simulink model "towTest_dualWinch"  (R2020a)
settings: Solver=FixedStepAuto  StartTime=0.0  StopTime=inf  FixedStep=Ts  RelTol=1e-3  EnableMultiTasking=on
undefined symbols (not defined in the file): encAng_trig, IO397, standard
libraries: xpcutilitieslib x52, hdlsllib x29, simulink x11, slrtlib x9, dspsigops x5, xpcseriallib x2, speedgoatlib_fpga_quadrature x2, powerlib_meascontrol x2, xpcrtudplib x2, speedgoatlib_fpga_dio x1, speedgoatlib_fpga_analog_io x1, speedgoatlib_IO581 x1
(part 1 of 2)
settings Model: Creator=MAE-VermillionLab  LastModifiedBy=MAE-VermillionLab
settings SolverCC: ConcurrentTasks=on  AutoInsertRateTranBlk=on
settings DataIOCC: SaveFormat=StructureWithTime
settings OptimizationCC: BlockReduction=off  OptimizeBlockIOStorage=off
settings HardwareCC: ProdBitPerPointer=32  ProdBitPerSizeT=32  ProdBitPerPtrDiffT=32  ProdLargestAtomicFloat=None  ProdWordSize=32  ProdLongLongMode=on  ProdHWDeviceType=Generic->32-bit x86 compatible
settings RTWCC: Description=Simulink Real-Time  SystemTargetFile=slrt.tlc  TLCOptions=-axPCMaxOverloads=30 -axPCOverLoadLen=2 -axPCStartupFlag=5  TemplateMakefile=slrt_default_tmf  CodeExecutionProfiling=on  RTWCompilerOptimization=on
settings SimulinkRealTimeCC: SupportVariableSizeSignals=on  RL32LogBufSizeModifier=1e8  xPCConcurrentTasks=on

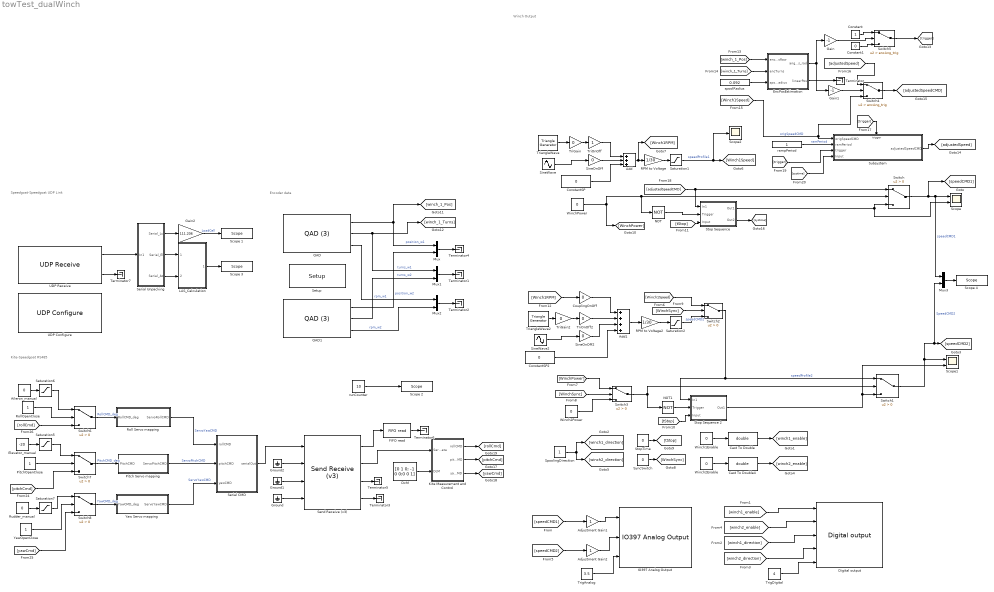
== system towTest_dualWinch ==
  note: Kite-Speedgoat RS485
  note: Speedgoat-Speedgoat UDP Link
  note: Winch Output
  note: Encoder data
  Add : Sum  Inputs=+++
  Add1 : Sum  Inputs=++++
  Adjustment Gain1 : Gain
  Adjustment Gain2 : Gain
  Aileron_manual : Constant  Value=0  OutDataTypeStr=int8
  Cast To Double : DataTypeConversion  OutDataTypeStr=double
  Cast To Double4 : DataTypeConversion  OutDataTypeStr=double
  Constant : Constant
  Constant1 : Constant  Value=0
  ConstantSP : Constant  Value=0
  ConstantSP2 : Constant  Value=0
  CouplingOnOff : Gain  Gain=0
  DcM : Constant  Value=[0 1 0; -1 0 0;0 0 1]
  Digital output : speedgoatlib_fpga_dio/Digital output  id=1  chan=[1:5]  init=[0]  reset=[0]  vectorizeInput=off  ts=Ts  pciSlot=-1  board=IO397-50k
      settings: SourceProductName=Simulink Real-Time: Speedgoat I/O Driver Library
  Elevator_manual : Constant  Value=-20  OutDataTypeStr=int8
  "EncPosEstimation " : Subsystem
  "FIFO read " : xpcseriallib/FIFO read   maxsize=1024  minsize=1  usedelimiter=off  delimiter=13  outputtype=8 bit uint null terminated  enable=off  enableout=off  sampletime=0.01
      settings: SourceProductBaseCode=XP
  Gain : Gain  Gain=-1
  Gain1 : Gain  Gain=-1
  Gain2 : Gain  Gain=111.206
  Ground : Ground
  Ground1 : Ground
  Ground2 : Ground
  IO397 Analog Output : speedgoatlib_fpga_analog_io/IO397 Analog Output  id=1  chan=[1:3]  initVal=0  resetVal=0  ts=Ts  pciSlot=-1  board=IO397-50k  span=+5 V
      settings: SourceProductName=Simulink Real-Time: Speedgoat I/O Driver Library
  "Kite Measurement and Control " : Subsystem
  LAS_Calculation : Subsystem
  Mux{,1..3} (4 alike) : Mux  Inputs=2
  NOT : Logic  Operator=NOT  IconShape=distinctive  AllPortsSameDT=off  OutDataTypeStr=boolean
  NOT1 : Logic  Operator=NOT  IconShape=distinctive  AllPortsSameDT=off  OutDataTypeStr=boolean
  "Pitch Servo mapping " : Subsystem
  PitchOpenClose : Constant
  QAD : speedgoatlib_fpga_quadrature/QAD (3)  id=1  board=IO397-50k  chan=[1]  resetOnStart=on  ts=Ts  pciSlot=-1  operatingMode=Quadrature decoder  indexControlMode=Ignore index  resolution=1x  stepsPerRevolution=[1800]  latchMode=Disabled  interpolatePosition=off  invertAB=off  showClearPositionInput=off  showClearIndexFoundInput=off  showPositionOutput=on  showTurnOutput=on  showSpeedOutput=on  showDirectionOutput=off  showIndexFoundOutput=off
      settings: SourceProductName=Simulink Real-Time: Speedgoat I/O Driver Library
  QAD1 : speedgoatlib_fpga_quadrature/QAD (3)  id=1  board=IO397-50k  chan=[2]  resetOnStart=on  ts=Ts  pciSlot=-1  operatingMode=Quadrature decoder  indexControlMode=Ignore index  resolution=1x  stepsPerRevolution=1800  latchMode=Disabled  interpolatePosition=off  invertAB=off  showClearPositionInput=off  showClearIndexFoundInput=off  showPositionOutput=on  showTurnOutput=on  showSpeedOutput=on  showDirectionOutput=off  showIndexFoundOutput=off
      settings: SourceProductName=Simulink Real-Time: Speedgoat I/O Driver Library
  RPM to Voltage : Gain  Gain=1/30
  RPM to Voltage2 : Gain  Gain=1/30
  Roll Servo mapping : Subsystem
  RollOpenClose : Constant
  Rudder_manual : Constant  Value=0  OutDataTypeStr=int8
  Saturation1 : Saturate  UpperLimit=5  LowerLimit=0
  Saturation2 : Saturate  UpperLimit=5  LowerLimit=0
  Saturation5 : Saturate  UpperLimit=30  LowerLimit=-30
  Saturation6 : Saturate  UpperLimit=30  LowerLimit=-30
  Saturation7 : Saturate  UpperLimit=30  LowerLimit=-30
  Scope : Scope  NumInputPorts=2
  Scope 1 : slrtlib/Displays and Logging/Scope   scopeno=6  scopetype=Target  autostart=on  viewmode=Numerical  formatstr='%15.6f'  grid=on  ylimits=[0,0]  nosamples=50  noprepostsamples=0  interleave=1  triggermode=FreeRun  triggersignal=1  trigsignalfromport=off  triggerlevel=0.0  triggerslope=Either  triggerscope=1  triggersample=0  filename=data.dat  mode=Lazy  writesize=512  autorestart=off  dynamicfilemode=off  maxwritefilesize=512*1024^2
  Scope 2 : slrtlib/Displays and Logging/Scope   scopeno=4  scopetype=Target  autostart=on  viewmode=Numerical  formatstr='%15.6f'  grid=on  ylimits=[0,0]  nosamples=50  noprepostsamples=0  interleave=1  triggermode=FreeRun  triggersignal=1  trigsignalfromport=off  triggerlevel=0.0  triggerslope=Either  triggerscope=1  triggersample=0  filename=data.dat  mode=Lazy  writesize=512  autorestart=off  dynamicfilemode=off  maxwritefilesize=512*1024^2
  Scope 3 : slrtlib/Displays and Logging/Scope   scopeno=5  scopetype=Target  autostart=on  viewmode=Numerical  formatstr='%15.6f'  grid=on  ylimits=[0,0]  nosamples=50  noprepostsamples=0  interleave=1  triggermode=FreeRun  triggersignal=1  trigsignalfromport=off  triggerlevel=0.0  triggerslope=Either  triggerscope=1  triggersample=0  filename=data.dat  mode=Lazy  writesize=512  autorestart=off  dynamicfilemode=off  maxwritefilesize=512*1024^2
  Scope 4 : slrtlib/Displays and Logging/Scope   scopeno=9  scopetype=Target  autostart=on  viewmode=Graphical sliding  formatstr='%15.6f'  grid=on  ylimits=[0,6]  nosamples=500  noprepostsamples=0  interleave=1  triggermode=FreeRun  triggersignal=1  trigsignalfromport=off  triggerlevel=0.0  triggerslope=Either  triggerscope=1  triggersample=0  filename=data.dat  mode=Lazy  writesize=512  autorestart=off  dynamicfilemode=off  maxwritefilesize=512*1024^2
  Scope1 : Scope  NumInputPorts=2
  Scope2 : Scope
  "Send Receive (v3) " : speedgoatlib_IO581/Send Receive (v3)   parModuleId=1  parSlot=-1  parModuleType=IO581  parTransceiver12=RS485 Half-Duplex  parTransceiver34=RS422  parTransceiver1=RS485 Half-Duplex  parAutoTurnaround1=off  parTurnaroundDelay1=0  parStandardBaud1=on  parBaudrate1=115200  parBaudDivisor1=1  parSamplingRate1=16x (standard)  parPrescale1=off  parCalcBaud1=7812500  parParity1=None  parDataBits1=8  parStopBits1=1  parTxTrigLvl1=1  parRxTrigLvl1=1  parHandshake1=none  parRtsHysteresis1=0  parXon1=17  parXoff1=19  parTxSwFifoSize1=1024  parTxSwFifoType1=8 bit uint null terminated  parRxSwFifoSize1=1024  parTransceiver2=RS485 Half-Duplex  parAutoTurnaround2=off  parTurnaroundDelay2=0  parStandardBaud2=on  parBaudrate2=115200  parBaudDivisor2=1  parSamplingRate2=16x (standard)  parPrescale2=off  parCalcBaud2=7812500  parParity2=None  parDataBits2=8  parStopBits2=1  parTxTrigLvl2=1  parRxTrigLvl2=1  parHandshake2=none  parRtsHysteresis2=0  parXon2=17  parXoff2=19  parTxSwFifoSize2=1024  parTxSwFifoType2=8 bit int null terminated  parRxSwFifoSize2=1024  parTransceiver3=RS422  parAutoTurnaround3=off  parTurnaroundDelay3=0  parStandardBaud3=on  parBaudrate3=115200  parBaudDivisor3=1  parSamplingRate3=16x (standard)  parPrescale3=off  parCalcBaud3=7812500  parParity3=None  parDataBits3=8  parStopBits3=1  parTxTrigLvl3=1  parRxTrigLvl3=8  parHandshake3=none  parRtsHysteresis3=0  parXon3=17  parXoff3=19  parTxSwFifoSize3=1024  parTxSwFifoType3=8 bit uint null terminated  parRxSwFifoSize3=1024  parTransceiver4=RS422  parAutoTurnaround4=off  parTurnaroundDelay4=0  parStandardBaud4=on  parBaudrate4=115200  parBaudDivisor4=1  parSamplingRate4=16x (standard)  parPrescale4=off  parCalcBaud4=7812500  parParity4=None  parDataBits4=8  parStopBits4=1  parTxTrigLvl4=1  parRxTrigLvl4=1  parHandshake4=none  parRtsHysteresis4=0  parXon4=17  parXoff4=19  parTxSwFifoSize4=1024  parTxSwFifoType4=8 bit uint null terminated  parRxSwFifoSize4=1024
      settings: SourceProductName=Simulink Real-Time: Speedgoat Library
  Serial CMD : Subsystem
  Serial Unpacking : Subsystem
  Setup : speedgoatlib_fpga/Setup/Setup  board=IO397-50k  id=1  device_id=1  frontIO=None  rearIO=None  bitstreamFile=init.mat  rev=1.0  timestamp_string=21/04/20 11:41:53  fpgaFreq=75 MHz  fpgaTick=13.33 ns  ProgSpiFlash=off  ProgBPIFlash=off  pciSlot=-1  PullRPort0=pull-up 3.3V  VioPort0=3.3V  PullRPort1=pull-up 3.3V  VioPort1=3.3V  PullRPort2=pull-up 3.3V  VioPort2=3.3V  PullRPort3=pull-up 3.3V  VioPort3=3.3V  PullRPort4=pull-up 3.3V  VioPort4=3.3V  PullRPort5=pull-up 3.3V  VioPort5=3.3V  PullRPort6=pull-up 3.3V  VioPort6=3.3V  PullRPort15=pull-up 3.3V  PullRPort31=pull-up 3.3V  PullRPort47=pull-up 3.3V  PullRPort63=pull-up 3.3V
      settings: SourceProductName=Simulink Real-Time: Speedgoat Library
  SineOnOff : Gain  Gain=0
  SineOnOff2 : Gain  Gain=0
  SineWave : Sin  Amplitude=0  Frequency=2*pi  SampleTime=0
  SineWave2 : Sin  Amplitude=0  Frequency=2*pi  SampleTime=0
  SpoolingDirection : Constant
  "Stop Sequence " : Subsystem
  Stop Sequence 2 : Subsystem
  StopTime : Constant  Value=0
  Subsystem : Subsystem
  Switch{,1..3,6..8} (7 alike) : Switch  Criteria=u2 > Threshold
  Switch4 : Switch  Criteria=u2 > Threshold  Threshold=encAng_trig
  Switch5 : Switch  Criteria=u2 > Threshold  Threshold=encAng_trig
  SyncSwitch : Constant  Value=0
  Terminator{,1..7} (8 alike) : Terminator
  TriGain : Gain  Gain=0
  TriGain2 : Gain  Gain=0
  TriOnOff : Gain
  TriOnOff2 : Gain  Gain=0
  TriangleWave : powerlib_meascontrol/Pulse & Signal Generators/Triangle Generator  Freq=1  Phase=90  Ts=0
  TriangleWave2 : powerlib_meascontrol/Pulse & Signal Generators/Triangle Generator  Freq=1  Phase=90  Ts=0
  TrigAnalog : Constant  Value=3.5
  TrigDigital : Constant  Value=4
  UDP Configure : xpcrtudplib/UDP Configure  Priority=-1  IpAddress=30.30.30.1  SubnetMask=255.255.255.0  Gateway=0.0.0.0  PciBus=15  PciSlot=0  PciFunction=0  ID=1  tune=0  disable=off  enableMulticast=off  MulticastIpAddress={}  MulticastMask={}
      settings: SourceProductBaseCode=XP
  UDP Receive : xpcrtudplib/UDP Receive  ipAddressVal=30.30.30.1  localPort=25001  rcvWidth=8  rcvFmAny=off  fmAddress=30.30.30.2  rcvMulticast=off  multicastAddress={}  maxUDPQueue=8  sampleTime=Ts
  Winch1Enable : Constant  Value=0
  Winch2Enable : Constant  Value=0
  Winch2Power : Constant  Value=0
  WinchPower : Constant  Value=0
  Yaw Servo mapping : Subsystem
  YawOpenClose : Constant
  rampPeriod : Constant
  runCounter : Constant  Value=10
  spoolRadius : Constant  Value=0.092
  wires:
  Switch/1 -> [speedCMD1], Mux3/1, Scope/1  "speedCMD1"
  WinchPower/1 -> NOT/1, Switch/2, [WinchPower]
  NOT/1 -> "Stop Sequence "/2(Trigger)
  Saturation1/1 -> Scope2/1, [Winch1Speed]  "speedProfile1"
  [speedCMD1] -> Adjustment Gain1/1
  Adjustment Gain1/1 -> IO397 Analog Output/1
  [winch1_enable] -> Digital output/1
  Cast To Double/1 -> [winch1_enable]
  Winch1Enable/1 -> Cast To Double/1
  ConstantSP/1 -> Add/3
  Add/1 -> [Winch1RPM], RPM to Voltage/1
  SineWave/1 -> SineOnOff/1
  [winch1_direction] -> Digital output/3
  Stop Sequence 2/1(Out1) -> Switch1/3, Scope1/2
  Switch1/1 -> Mux3/2, [speedCMD2], Scope1/1  "SpeedCMD2"
  SpoolingDirection/1 -> [winch1_direction], [winch2_direction]
  Switch3/1 -> NOT1/1, Switch1/2
  Cast To Double4/1 -> [winch2_enable]
  Winch2Enable/1 -> Cast To Double4/1
  Switch2/1 -> Stop Sequence 2/1(In1), Switch1/1  "speedProfile2"
  Adjustment Gain2/1 -> IO397 Analog Output/2
  [speedCMD2] -> Adjustment Gain2/1
  [winch2_enable] -> Digital output/2
  [winch2_direction] -> Digital output/4
  TriangleWave/1 -> TriGain/1
  TriGain/1 -> TriOnOff/1
  TriOnOff/1 -> Add/1
  SineOnOff/1 -> Add/2
  RPM to Voltage/1 -> Saturation1/1
  TriangleWave2/1 -> TriGain2/1
  RPM to Voltage2/1 -> Saturation2/1
  Add1/1 -> RPM to Voltage2/1
  SineWave2/1 -> SineOnOff2/1
  TriGain2/1 -> TriOnOff2/1
  TriOnOff2/1 -> Add1/2
  SineOnOff2/1 -> Add1/3
  Saturation2/1 -> Switch2/3  "speedCMD2"
  [Winch1Speed] -> Switch2/1
  SyncSwitch/1 -> [WinchSync]
  [WinchSync] -> Switch2/2
  "Stop Sequence "/1(Out1) -> Scope/2, Switch/3
  StopTime/1 -> [tStop]
  [tStop] -> "Stop Sequence "/3(Input)
  [tStop] -> Stop Sequence 2/3(Input)
  NOT1/1 -> Stop Sequence 2/2(Trigger)
  [WinchPower] -> Switch3/1
  Winch2Power/1 -> Switch3/3
  [WinchSync] -> Switch3/2
  [Winch1RPM] -> CouplingOnOff/1
  ConstantSP2/1 -> Add1/4
  CouplingOnOff/1 -> Add1/1
  QAD1/1 -> Mux/2  "position_w2"
  QAD/1 -> [winch_1_Pos], Mux/1  "position_w1"
  QAD/2 -> [winch_1_Turns], Mux1/1  "turns_w1"
  QAD1/2 -> Mux1/2  "turns_w2"
  QAD/3 -> Mux2/1  "rpm_w1"
  QAD1/3 -> Mux2/2  "rpm_w2"
  Mux3/1 -> Scope 4/1
  [winch_1_Pos] -> "EncPosEstimation "/1(encPosRaw)
  [winch_1_Turns] -> "EncPosEstimation "/2(encTurns)
  spoolRadius/1 -> "EncPosEstimation "/3(spoolRadius)
  "EncPosEstimation "/2(linearPos) -> Terminator/1
  "EncPosEstimation "/1(angPos_rad) -> Gain/1, Gain1/1
  [Winch1Speed] -> Switch4/3, Subsystem/1(origSpeedCMD)  "origSpeedCMD"
  Constant/1 -> Switch5/1
  Constant1/1 -> Switch5/3
  rampPeriod/1 -> Subsystem/2(ramPeriod)  "ramPeriod"
  Subsystem/1(adjustedSpeedCMD) -> [adjustedSpeed]
  [trigger] -> Subsystem/Trigger
  [adjustedSpeedCMD] -> "Stop Sequence "/1(In1), Switch/1
  Switch4/1 -> [adjustedSpeedCMD]
  Gain/1 -> Switch5/2
  Gain1/1 -> Switch4/2
  [adjustedSpeed] -> Switch4/1
  Switch5/1 -> [trigger]
  [trigger] -> Subsystem/3(trigger)
  "Stop Sequence "/2(Out2) -> [systime]
  [systime] -> Subsystem/4(Input)
  Mux1/1 -> Terminator1/1
  Mux2/1 -> Terminator2/1
  Mux/1 -> Terminator4/1
  DcM/1 -> "Kite Measurement and Control "/2(DcM)
  Serial CMD/1(serialOut) -> "Send Receive (v3) "/1
  "Kite Measurement and Control "/1(rollCMD) -> [rollCmd]
  "Send Receive (v3) "/2 -> "Kite Measurement and Control "/1(SerialData)
  "Send Receive (v3) "/1 -> "FIFO read "/1
  Ground2/1 -> "Send Receive (v3) "/2
  "Kite Measurement and Control "/3(yawCMD) -> [yawCmd]
  Ground1/1 -> "Send Receive (v3) "/3
  "FIFO read "/1 -> Terminator6/1
  "Kite Measurement and Control "/2(pitchCMD) -> [pitchCmd]
  Ground/1 -> "Send Receive (v3) "/4
  "Send Receive (v3) "/4 -> Terminator3/1
  "Send Receive (v3) "/3 -> Terminator5/1
  Serial Unpacking/2(Serial_El) -> LAS_Calculation/1(Serial_El)
  UDP Receive/2 -> Terminator7/1
  Serial Unpacking/3(Serial_Az) -> LAS_Calculation/2(Serial_Az)
  UDP Receive/1 -> Serial Unpacking/1(In1)
  Serial Unpacking/1(Serial_Lc) -> Gain2/1
  LAS_Calculation/1(Output) -> Scope 3/1
  Gain2/1 -> Scope 1/1  "LoadCell"
  "Pitch Servo mapping "/1(ServoPitchCMD) -> Serial CMD/2(pitchCMD)  "ServoPitchCMD"
  Yaw Servo mapping/1(ServoYawCMD) -> Serial CMD/3(yawCMD)  "ServoYawCMD"
  Roll Servo mapping/1(ServoRollCMD) -> Serial CMD/1("rollCMD ")  "ServoYawCMD"
  [rollCmd] -> Switch6/3
  [yawCmd] -> Switch8/3
  Aileron_manual/1 -> Saturation6/1
  [pitchCmd] -> Switch7/3
  Elevator_manual/1 -> Saturation5/1
  Saturation6/1 -> Switch6/1
  Switch8/1 -> Yaw Servo mapping/1(YawCMD_deg)  "YawCMD_deg"
  Switch6/1 -> Roll Servo mapping/1(RollCMD_deg)  "RollCMD_deg"
  RollOpenClose/1 -> Switch6/2
  Rudder_manual/1 -> Saturation7/1
  Switch7/1 -> "Pitch Servo mapping "/1(PitchCMD)  "PitchCMD_deg"
  Saturation7/1 -> Switch8/1
  PitchOpenClose/1 -> Switch7/2
  YawOpenClose/1 -> Switch8/2
  Saturation5/1 -> Switch7/1
  TrigAnalog/1 -> IO397 Analog Output/3
  TrigDigital/1 -> Digital output/5
  runCounter/1 -> Scope 2/1

== system towTest_dualWinch/EncPosEstimation  ==
  encPosRaw : Inport
  encTurns : Inport  Port=2
  spoolRadius : Inport  Port=3
  Add1 : Sum
  Cast To Double : DataTypeConversion  OutDataTypeStr=double
  Gain : Gain  Gain=(2*pi)/1800
  Gain1 : Gain  Gain=1800
  Product : Product
  angPos_rad : Outport
  linearPos : Outport  Port=2
  wires:
  Gain/1 -> angPos_rad/1, Product/1  "angPos_rad"
  Cast To Double/1 -> Add1/1
  Add1/1 -> Gain/1
  Gain1/1 -> Add1/2
  Product/1 -> linearPos/1  "linearPos"
  encTurns/1 -> Gain1/1
  spoolRadius/1 -> Product/2
  encPosRaw/1 -> Cast To Double/1

== system towTest_dualWinch/Kite Measurement and Control  ==
  SerialData : Inport
  DcM : Inport  Port=2
  Bus Selector : BusSelector  OutputSignals=rollCmd,pitchCmd,yawCmd
  Controller1 : Subsystem  mask{ctrlSurfDefMax=45, pitchKP=1, yawKP=1, rollKP=1}
      mask prompts: ctrlSurfDefMax "Max Ctrlsurf def"; pitchKP "pitch Kp"; yawKP "yaw Kp"; rollKP "roll Kp"
  "Euler setpoints " : Subsystem  mask{EulerSP=[0 0 0]}
      mask prompts: EulerSP "Euler Setpoints"
  "Kite Measurements " : Subsystem
  rollCMD : Outport
  pitchCMD : Outport  Port=2
  yawCMD : Outport  Port=3
  wires:
  "Kite Measurements "/1(kiteMeasure) -> Controller1/2(kiteMeasure)  "kiteMeasure"
  Bus Selector/3 -> yawCMD/1  "<yawCmd>"
  Controller1/1(Cmd) -> Bus Selector/1
  Bus Selector/2 -> pitchCMD/1  "<pitchCmd>"
  Bus Selector/1 -> rollCMD/1  "<rollCmd>"
  SerialData/1 -> "Kite Measurements "/1(In1)
  DcM/1 -> "Kite Measurements "/2(Input)
  "Euler setpoints "/1(setPoints) -> Controller1/1(setPoints)  "setPoints"

== system towTest_dualWinch/LAS_Calculation ==
  Serial_El : Inport
  Serial_Az : Inport  Port=2
  Add2 : Sum
  Add3 : Sum
  Az_deg_calib : Constant  Value=-343.5468
  Constant : Constant  Value=360
  Constant2 : Constant  Value=360
  El_deg_calib : Constant  Value=-243.544
  Gain : Gain  Gain=360/8192
  Gain1 : Gain  Gain=360/8192
  Gain2 : Gain  Gain=pi/180
  Gain3 : Gain  Gain=pi/180
  Gain4 : Gain  Gain=180/pi
  Gain5 : Gain  Gain=180/pi
  LAS Measurement Corrections : MATLAB Function  TreatAsAtomicUnit=on
  Mod : Math  Operator=mod  SaturateOnIntegerOverflow=on
  Mod1 : Math  Operator=mod  SaturateOnIntegerOverflow=on
  Mux : Mux
  ifOutsideBounds : MATLAB Function  TreatAsAtomicUnit=on
  ifOutsideBounds1 : MATLAB Function  TreatAsAtomicUnit=on
  Output : Outport
  wires:
  Gain/1 -> Mod/1
  Constant2/1 -> Mod1/2
  Constant/1 -> Mod/2
  Mod/1 -> Add2/1
  Serial_Az/1 -> Gain1/1
  Mod1/1 -> Add3/1
  Gain1/1 -> Mod1/1
  ifOutsideBounds/1(y) -> Mux/3, Gain2/1  "El_deg"
  Add3/1 -> ifOutsideBounds1/1(u)  "Az_deg"
  Serial_El/1 -> Gain/1  "Elevation"
  Gain2/1 -> LAS Measurement Corrections/1(elev_encoder)
  Gain3/1 -> LAS Measurement Corrections/2(azi_encoder)
  LAS Measurement Corrections/2(azi) -> Gain5/1
  LAS Measurement Corrections/1(elev) -> Gain4/1
  Gain4/1 -> Mux/1  "kite_elev"
  Gain5/1 -> Mux/2  "kite_azi"
  Mux/1 -> Output/1
  Az_deg_calib/1 -> Add3/2
  El_deg_calib/1 -> Add2/2
  Add2/1 -> ifOutsideBounds/1(u)  "El_deg"
  ifOutsideBounds1/1(y) -> Gain3/1, Mux/4  "Az_deg"

== system towTest_dualWinch/Pitch Servo mapping  ==
  note: Negative gain added due to servo orientation
  PitchCMD : Inport
  Add2 : Sum
  Add3 : Sum
  "Bias " : Constant  Value=7.2
  Constant2 : Constant  Value=-0.2065
  Display : Display
  Display1 : Display
  Gain3 : Gain  Gain=2.732
  Gain4 : Gain  Gain=-1
  ServoPitchCMD : Outport
  wires:
  Add2/1 -> Add3/1
  Constant2/1 -> Add2/2
  Gain4/1 -> Gain3/1
  "Bias "/1 -> Add3/2  "PitchServoBias"
  Add3/1 -> Display/1, ServoPitchCMD/1
  PitchCMD/1 -> Display1/1, Gain4/1
  Gain3/1 -> Add2/1

== system towTest_dualWinch/Roll Servo mapping ==
  RollCMD_deg : Inport
  Add2 : Sum
  Bias : Constant  Value=0
  ServoRollCMD : Outport
  wires:
  Bias/1 -> Add2/2  "RollServoBias"
  RollCMD_deg/1 -> Add2/1
  Add2/1 -> ServoRollCMD/1

== system towTest_dualWinch/Serial CMD ==
  note: Subsystem
  "rollCMD " : Inport
  pitchCMD : Inport  Port=2
  yawCMD : Inport  Port=3
  Constant : Constant  Value=0x11  OutDataTypeStr=uint8
  Constant1 : Constant  Value=0x01  OutDataTypeStr=uint8
  Mux : Mux  Inputs=8
  Mux1 : Mux  Inputs=3
  Mux2 : Mux  Inputs=3
  Mux3 : Mux  Inputs=3
  Scope 1 : slrtlib/Displays and Logging/Scope   scopeno=3  scopetype=Target  autostart=on  viewmode=Graphical sliding  formatstr='%15.6f'  grid=on  ylimits=[-60,60]  nosamples=500  noprepostsamples=0  interleave=1  triggermode=FreeRun  triggersignal=1  trigsignalfromport=off  triggerlevel=0.0  triggerslope=Either  triggerscope=1  triggersample=0  filename=data.dat  mode=Lazy  writesize=512  autorestart=off  dynamicfilemode=off  maxwritefilesize=512*1024^2
  Scope 2 : slrtlib/Displays and Logging/Scope   scopeno=7  scopetype=Target  autostart=on  viewmode=Numerical  formatstr='%15.6f'  grid=on  ylimits=[0,100]  nosamples=50  noprepostsamples=0  interleave=1  triggermode=FreeRun  triggersignal=1  trigsignalfromport=off  triggerlevel=0.0  triggerslope=Either  triggerscope=1  triggersample=0  filename=data.dat  mode=Lazy  writesize=512  autorestart=off  dynamicfilemode=off  maxwritefilesize=512*1024^2
  Scope 3 : slrtlib/Displays and Logging/Scope   scopeno=8  scopetype=Target  autostart=on  viewmode=Numerical  formatstr='%15.6f'  grid=on  ylimits=[0,100]  nosamples=50  noprepostsamples=0  interleave=1  triggermode=FreeRun  triggersignal=1  trigsignalfromport=off  triggerlevel=0.0  triggerslope=Either  triggerscope=1  triggersample=0  filename=data.dat  mode=Lazy  writesize=512  autorestart=off  dynamicfilemode=off  maxwritefilesize=512*1024^2
  deg-to-us : Subsystem
  deg-to-us1 : Subsystem
  deg-to-us2 : Subsystem
  to2uint1 : Subsystem
  to2uint2 : Subsystem
  to2uint8 : Subsystem
  serialOut : Outport
  wires:
  pitchCMD/1 -> deg-to-us1/1(pitchCMD), Mux2/2, Mux1/2  "pitchCMD"
  Constant/1 -> Mux/2
  to2uint8/1(Out1) -> Mux/3
  to2uint8/2(Out2) -> Mux/4
  yawCMD/1 -> Mux1/3, deg-to-us2/1(In1), Mux2/3  "yawCMD"
  Mux/1 -> serialOut/1
  Mux1/1 -> Scope 1/1
  "rollCMD "/1 -> Mux1/1, deg-to-us/1(In1), Mux2/1  "rollCMD"
  to2uint1/1(Out1) -> Mux/5
  to2uint1/2(Out2) -> Mux/6
  to2uint2/1(Out1) -> Mux/7
  to2uint2/2(Out2) -> Mux/8
  deg-to-us1/1(Out1) -> to2uint1/1(" "), Mux3/2
  deg-to-us2/1(Out1) -> to2uint2/1(" "), Mux3/3
  Mux2/1 -> Scope 2/1
  Mux3/1 -> Scope 3/1
  deg-to-us/1(Out1) -> to2uint8/1(" "), Mux3/1
  Constant1/1 -> Mux/1

== system towTest_dualWinch/Serial Unpacking ==
  In1 : Inport
  Demux : Demux  Outputs=8
  Display2 : Display
  Display7 : Display
  Display8 : Display
  Subsystem : Subsystem
  Subsystem1 : Subsystem
  binary2double5 : Subsystem
  Serial_Lc : Outport
  Serial_El : Outport  Port=2
  Serial_Az : Outport  Port=3
  wires:
  Demux/6 -> Subsystem/2(In2)
  Demux/5 -> Subsystem/1(In1)
  In1/1 -> Demux/1
  Subsystem/1(Double) -> Display7/1, Serial_El/1
  Demux/8 -> Subsystem1/2(In2)
  Demux/7 -> Subsystem1/1(In1)
  Subsystem1/1(Double) -> Display8/1, Serial_Az/1
  Demux/1 -> binary2double5/1(In1)
  Demux/2 -> binary2double5/2(In2)
  Demux/3 -> binary2double5/3(In3)
  Demux/4 -> binary2double5/4(In4)
  binary2double5/1(Double) -> Display2/1, Serial_Lc/1  "Yaw Rate"

== system towTest_dualWinch/Stop Sequence  ==
  In1 : Inport
  Trigger : Inport  Port=2
  Input : Inport  Port=3
  Add : Sum  Inputs=-+
  Add1 : Sum  Inputs=+-
  Clock : Clock
  Divide : Product  Inputs=**/
  Sample and Hold : dspsigops/Sample and Hold  trig=Rising edge  initCond=0  latchinput=off
  Sample and Hold1 : dspsigops/Sample and Hold  trig=Rising edge  initCond=0  latchinput=off
  Saturation : Saturate  UpperLimit=5  LowerLimit=0
  Out1 : Outport
  Out2 : Outport  Port=2
  wires:
  Trigger/1 -> Sample and Hold1/Trigger, Sample and Hold/Trigger
  Add/1 -> Divide/2
  In1/1 -> Sample and Hold/1
  Divide/1 -> Add1/2
  Sample and Hold/1 -> Divide/1, Add1/1
  Sample and Hold1/1 -> Add/1
  Clock/1 -> Out2/1, Add/2, Sample and Hold1/1
  Add1/1 -> Saturation/1
  Saturation/1 -> Out1/1
  Input/1 -> Divide/3

== system towTest_dualWinch/Stop Sequence 2 ==
  In1 : Inport
  Trigger : Inport  Port=2
  Input : Inport  Port=3
  Add : Sum  Inputs=-+
  Add1 : Sum  Inputs=+-
  Clock : Clock
  Divide : Product  Inputs=**/
  Sample and Hold : dspsigops/Sample and Hold  trig=Rising edge  initCond=0  latchinput=off
  Sample and Hold1 : dspsigops/Sample and Hold  trig=Rising edge  initCond=0  latchinput=off
  Saturation : Saturate  UpperLimit=5  LowerLimit=0
  Out1 : Outport
  wires:
  Input/1 -> Divide/3
  Saturation/1 -> Out1/1
  Add1/1 -> Saturation/1
  Clock/1 -> Sample and Hold1/1, Add/2
  Sample and Hold1/1 -> Add/1
  Sample and Hold/1 -> Add1/1, Divide/1
  Divide/1 -> Add1/2
  In1/1 -> Sample and Hold/1
  Add/1 -> Divide/2
  Trigger/1 -> Sample and Hold/Trigger, Sample and Hold1/Trigger

== system towTest_dualWinch/Subsystem ==
  origSpeedCMD : Inport
  ramPeriod : Inport  Port=2
  trigger : Inport  Port=3
  Input : Inport  Port=4
  Trigger : TriggerPort  VariantControl=Variant  PortDimensions=1
  Add : Sum  Inputs=+-
  Add2 : Sum
  Divide : Product  Inputs=*/
  Gain : Gain  Gain=0.08
  Gain1 : Gain  Gain=1.08
  Product : Product
  Sample and Hold : dspsigops/Sample and Hold  trig=Rising edge  initCond=0  latchinput=off
  Saturation Dynamic : simulink/Discontinuities/Saturation Dynamic  OutMin=[]  OutMax=[]  OutDataTypeStr=Inherit: Same as second input  OutDataType=fixdt(1, 16)  OutScaling=2^-10  RndMeth=Zero  DoSatur=off
  adjustedSpeedCMD : Outport
  wires:
  Saturation Dynamic/1 -> adjustedSpeedCMD/1  "adjustedSpeedCMD"
  origSpeedCMD/1 -> [Winch1Speed], Gain/1
  Gain/1 -> Divide/1
  [Winch1Speed] -> Gain1/1, Saturation Dynamic/3  "origSpeedCMD"
  [Winch1Speed] -> Add2/2  "origSpeedCMD"
  Gain1/1 -> Saturation Dynamic/1
  ramPeriod/1 -> Divide/2
  Add2/1 -> Saturation Dynamic/2
  Input/1 -> [time], Sample and Hold/1
  trigger/1 -> Sample and Hold/Trigger
  Sample and Hold/1 -> [triggerTime]
  [time] -> Add/1
  [triggerTime] -> Add/2
  Divide/1 -> Product/2
  Add/1 -> Product/1
  Product/1 -> Add2/1

== system towTest_dualWinch/Yaw Servo mapping ==
  YawCMD_deg : Inport
  Add2 : Sum
  Bias : Constant  Value=0
  ServoYawCMD : Outport
  wires:
  Bias/1 -> Add2/2  "YawServoBias"
  YawCMD_deg/1 -> Add2/1
  Add2/1 -> ServoYawCMD/1

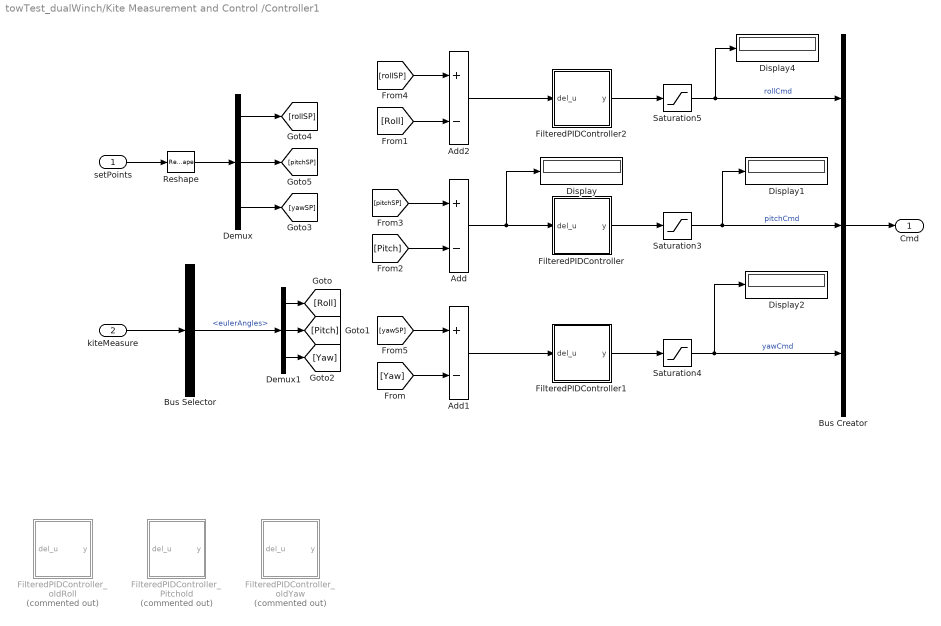
== system towTest_dualWinch/Kite Measurement and Control /Controller1 ==
  setPoints : Inport
  kiteMeasure : Inport  Port=2
  Add : Sum  Inputs=+-
  Add1 : Sum  Inputs=+-
  Add2 : Sum  Inputs=+-
  Bus Creator : BusCreator  Inputs=3
  Bus Selector : BusSelector  OutputSignals=eulerAngles
  Demux : Demux  Outputs=3
  Demux1 : Demux  Outputs=3
  Display{,1..2,4} (4 alike) : Display
  FilteredPIDController : Subsystem  mask{Kp=1, Kd=0, tau=1, Ki=0}
      mask prompts: Kp "Proportional Gain"; Kd "Derivative Gain"; tau "Time constant"; Ki "Integral Gain"
  FilteredPIDController1 : Subsystem  mask{Kp=1, Kd=0, tau=1, Ki=0}
      mask prompts: Kp "Proportional Gain"; Kd "Derivative Gain"; tau "Time constant"; Ki "Integral Gain"
  FilteredPIDController2 : Subsystem  mask{Kp=1, Kd=0, tau=1, Ki=0}
      mask prompts: Kp "Proportional Gain"; Kd "Derivative Gain"; tau "Time constant"; Ki "Integral Gain"
  FilteredPIDController_Pitchold : Subsystem  Commented=on  mask{Kp=1, Kd=0, tau=1, Ki=0}
      mask prompts: Kp "Proportional Gain"; Kd "Derivative Gain"; tau "Time constant"; Ki "Integral Gain"
  FilteredPIDController_oldRoll : Subsystem  Commented=on  mask{Kp=1, Kd=0, tau=1, Ki=0}
      mask prompts: Kp "Proportional Gain"; Kd "Derivative Gain"; tau "Time constant"; Ki "Integral Gain"
  FilteredPIDController_oldYaw : Subsystem  Commented=on  mask{Kp=1, Kd=0, tau=1, Ki=0}
      mask prompts: Kp "Proportional Gain"; Kd "Derivative Gain"; tau "Time constant"; Ki "Integral Gain"
  Reshape : Reshape  OutputDimensionality=Column vector (2-D)
  Saturation3 : Saturate  UpperLimit=30  LowerLimit=-30
  Saturation4 : Saturate  UpperLimit=30  LowerLimit=-30
  Saturation5 : Saturate  UpperLimit=30  LowerLimit=-30
  Cmd : Outport
  wires:
  [Pitch] -> Add/2
  [Yaw] -> Add1/2
  [yawSP] -> Add1/1
  Demux/3 -> [yawSP]
  [pitchSP] -> Add/1
  kiteMeasure/1 -> Bus Selector/1
  Saturation4/1 -> Display2/1, Bus Creator/3  "yawCmd"
  Saturation5/1 -> Display4/1, Bus Creator/1  "rollCmd"
  Bus Creator/1 -> Cmd/1
  Reshape/1 -> Demux/1
  setPoints/1 -> Reshape/1
  Add/1 -> FilteredPIDController/1(del_u), Display/1
  [rollSP] -> Add2/1
  [Roll] -> Add2/2
  Demux/2 -> [pitchSP]
  Demux/1 -> [rollSP]
  Bus Selector/1 -> Demux1/1  "<eulerAngles>"
  Demux1/1 -> [Roll]
  Demux1/2 -> [Pitch]
  Demux1/3 -> [Yaw]
  Saturation3/1 -> Display1/1, Bus Creator/2  "pitchCmd"
  FilteredPIDController/1(y) -> Saturation3/1
  FilteredPIDController2/1(y) -> Saturation5/1
  Add2/1 -> FilteredPIDController2/1(del_u)
  FilteredPIDController1/1(y) -> Saturation4/1
  Add1/1 -> FilteredPIDController1/1(del_u)

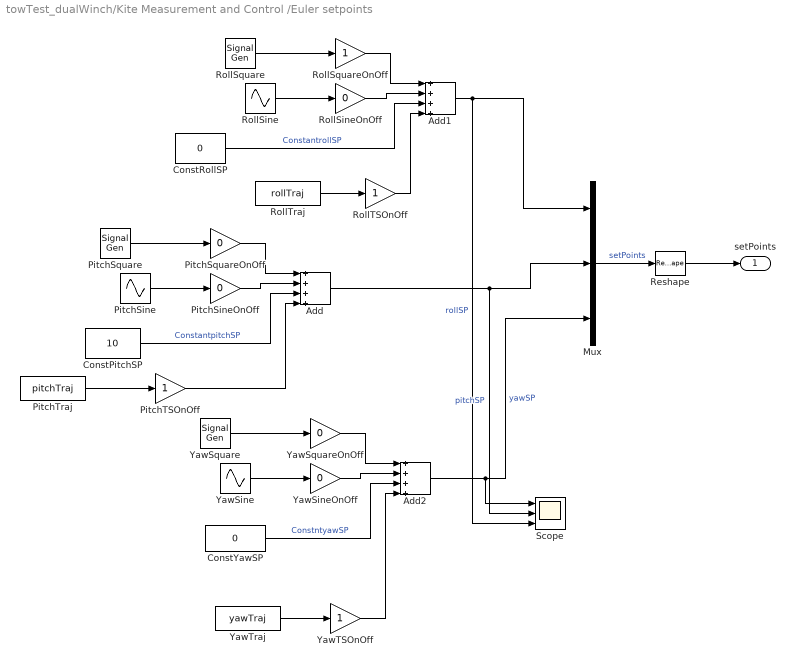
== system towTest_dualWinch/Kite Measurement and Control /Euler setpoints  ==
  Add : Sum  Inputs=++++
  Add1 : Sum  Inputs=++++
  Add2 : Sum  Inputs=++++
  ConstPitchSP : Constant  Value=10
  ConstRollSP : Constant  Value=0
  ConstYawSP : Constant  Value=0
  Mux : Mux  Inputs=3
  PitchSine : Sin  Amplitude=20  Frequency=1.5708  SampleTime=0
  PitchSineOnOff : Gain  Gain=0
  PitchSquare : SignalGenerator  WaveForm=square  Amplitude=20  Frequency=1.5708  Units=rad/sec
  PitchSquareOnOff : Gain  Gain=0
  PitchTSOnOff : Gain
  PitchTraj : FromWorkspace  VariableName=pitchTraj
  Reshape : Reshape  OutputDimensionality=Column vector (2-D)
  RollSine : Sin  Amplitude=10  Frequency=2.0944  SampleTime=0
  RollSineOnOff : Gain  Gain=0
  RollSquare : SignalGenerator  WaveForm=square  Amplitude=10  Frequency=1.0472  Units=rad/sec
  RollSquareOnOff : Gain
  RollTSOnOff : Gain
  RollTraj : FromWorkspace  VariableName=rollTraj
  Scope : Scope  NumInputPorts=3
  YawSine : Sin  Amplitude=15  Frequency=3.1416  SampleTime=0
  YawSineOnOff : Gain  Gain=0
  YawSquare : SignalGenerator  WaveForm=square  Amplitude=10  Units=rad/sec
  YawSquareOnOff : Gain  Gain=0
  YawTSOnOff : Gain
  YawTraj : FromWorkspace  VariableName=yawTraj
  setPoints : Outport
  wires:
  Mux/1 -> Reshape/1  "setPoints"
  Reshape/1 -> setPoints/1
  PitchSineOnOff/1 -> Add/2
  PitchSine/1 -> PitchSineOnOff/1
  PitchSquareOnOff/1 -> Add/1
  PitchSquare/1 -> PitchSquareOnOff/1
  ConstPitchSP/1 -> Add/3  "ConstantpitchSP"
  RollSineOnOff/1 -> Add1/2
  RollSquareOnOff/1 -> Add1/1
  RollSine/1 -> RollSineOnOff/1
  RollSquare/1 -> RollSquareOnOff/1
  ConstRollSP/1 -> Add1/3  "ConstantrollSP"
  YawSineOnOff/1 -> Add2/2
  YawSquareOnOff/1 -> Add2/1
  YawSine/1 -> YawSineOnOff/1
  YawSquare/1 -> YawSquareOnOff/1
  ConstYawSP/1 -> Add2/3  "ConstntyawSP"
  Add2/1 -> Scope/1, Mux/3  "yawSP"
  Add/1 -> Scope/2, Mux/2  "pitchSP"
  Add1/1 -> Scope/3, Mux/1  "rollSP"
  RollTSOnOff/1 -> Add1/4
  RollTraj/1 -> RollTSOnOff/1
  PitchTSOnOff/1 -> Add/4
  YawTSOnOff/1 -> Add2/4
  PitchTraj/1 -> PitchTSOnOff/1
  YawTraj/1 -> YawTSOnOff/1

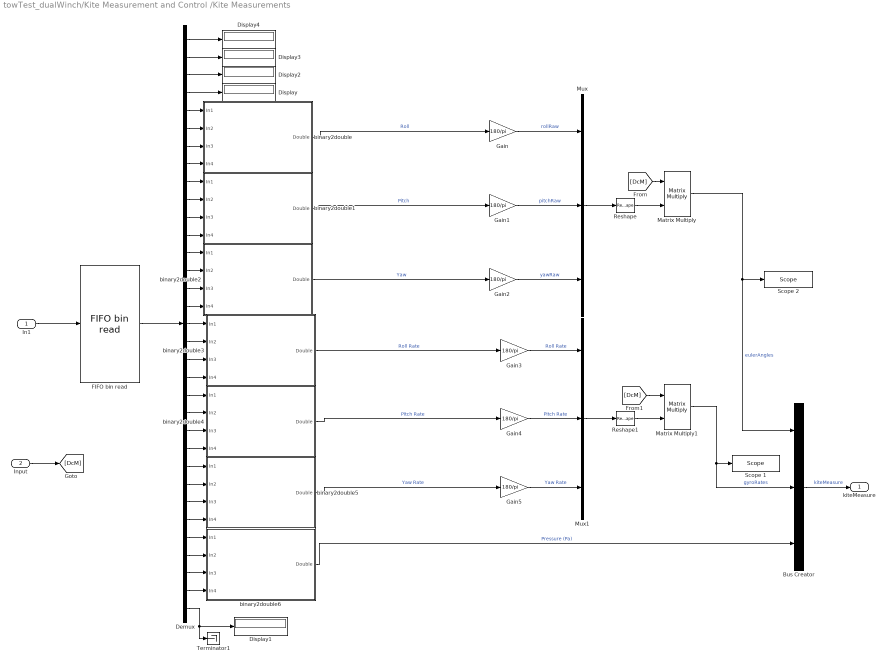
== system towTest_dualWinch/Kite Measurement and Control /Kite Measurements  ==
  In1 : Inport
  Input : Inport  Port=2
  Bus Creator : BusCreator  Inputs=3
  Demux : Demux  Outputs=33
  Display{,1..4} (5 alike) : Display
      Display settings: Format=hex (Stored Integer)
      Display2 settings: Format=hex (Stored Integer)
      Display3 settings: Format=hex (Stored Integer)
      Display4 settings: Format=hex (Stored Integer)
  "FIFO bin read " : xpcseriallib/FIFO bin read   header={[0x47 0xBB 0x3C 0x2B]}  lengths=[32]  hold=Hold last output if no new data  enable=off  maxsize=32  outputtype=8 bit uint null terminated  sampletime=0.01
      settings: SourceProductBaseCode=XP
  Gain{,1..5} (6 alike) : Gain  Gain=180/pi
  Matrix Multiply : Product  Multiplication=Matrix(*)
  Matrix Multiply1 : Product  Multiplication=Matrix(*)
  Mux : Mux  Inputs=3
  Mux1 : Mux  Inputs=3
  Reshape : Reshape  OutputDimensionality=Column vector (2-D)
  Reshape1 : Reshape  OutputDimensionality=Column vector (2-D)
  Scope 1 : slrtlib/Displays and Logging/Scope   scopeno=2  scopetype=Target  autostart=on  viewmode=Graphical sliding  formatstr='%15.6f'  grid=on  ylimits=[-100,100]  nosamples=500  noprepostsamples=0  interleave=1  triggermode=FreeRun  triggersignal=1  trigsignalfromport=off  triggerlevel=0.0  triggerslope=Either  triggerscope=1  triggersample=0  filename=data.dat  mode=Lazy  writesize=512  autorestart=off  dynamicfilemode=off  maxwritefilesize=512*1024^2
  Scope 2 : slrtlib/Displays and Logging/Scope   scopeno=1  scopetype=Target  autostart=on  viewmode=Graphical sliding  formatstr='%15.6f'  grid=on  ylimits=[-100,100]  nosamples=500  noprepostsamples=0  interleave=1  triggermode=FreeRun  triggersignal=1  trigsignalfromport=off  triggerlevel=0.0  triggerslope=Either  triggerscope=1  triggersample=0  filename=data.dat  mode=Lazy  writesize=512  autorestart=off  dynamicfilemode=off  maxwritefilesize=512*1024^2
  Terminator1 : Terminator
  binary2double : Subsystem
  binary2double1 : Subsystem
  binary2double2 : Subsystem
  binary2double3 : Subsystem
  binary2double4 : Subsystem
  binary2double5 : Subsystem
  binary2double6 : Subsystem
  kiteMeasure : Outport
  wires:
  binary2double/1(Double) -> Gain/1  "Roll"
  binary2double1/1(Double) -> Gain1/1  "Pitch"
  binary2double5/1(Double) -> Gain5/1  "Yaw Rate"
  binary2double6/1(Double) -> Bus Creator/3  "Pressure (Pa)"
  binary2double4/1(Double) -> Gain4/1  "Pitch Rate"
  binary2double3/1(Double) -> Gain3/1  "Roll Rate"
  binary2double2/1(Double) -> Gain2/1  "Yaw"
  Bus Creator/1 -> kiteMeasure/1  "kiteMeasure"
  Demux/28 -> binary2double5/4(In4)
  Demux/31 -> binary2double6/3(In3)
  Demux/13 -> binary2double2/1(In1)
  Demux/23 -> binary2double4/3(In3)
  Demux/21 -> binary2double4/1(In1)
  Demux/16 -> binary2double2/4(In4)
  Demux/33 -> Terminator1/1, Display1/1
  Demux/11 -> binary2double1/3(In3)
  Demux/22 -> binary2double4/2(In2)
  Demux/29 -> binary2double6/1(In1)
  Demux/19 -> binary2double3/3(In3)
  Demux/9 -> binary2double1/1(In1)
  Demux/7 -> binary2double/3(In3)
  In1/1 -> "FIFO bin read "/1
  Demux/10 -> binary2double1/2(In2)
  Demux/8 -> binary2double/4(In4)
  Demux/6 -> binary2double/2(In2)
  Demux/12 -> binary2double1/4(In4)
  Demux/14 -> binary2double2/2(In2)
  Demux/4 -> Display/1
  Demux/17 -> binary2double3/1(In1)
  Demux/18 -> binary2double3/2(In2)
  Demux/30 -> binary2double6/2(In2)
  Demux/25 -> binary2double5/1(In1)
  Demux/15 -> binary2double2/3(In3)
  Demux/5 -> binary2double/1(In1)
  Demux/26 -> binary2double5/2(In2)
  Demux/20 -> binary2double3/4(In4)
  Demux/32 -> binary2double6/4(In4)
  Demux/27 -> binary2double5/3(In3)
  Demux/24 -> binary2double4/4(In4)
  "FIFO bin read "/1 -> Demux/1
  Gain2/1 -> Mux/3  "yawRaw"
  Gain1/1 -> Mux/2  "pitchRaw"
  Gain/1 -> Mux/1  "rollRaw"
  Input/1 -> [DcM]
  Mux/1 -> Reshape/1
  Gain3/1 -> Mux1/1  "Roll Rate"
  Gain4/1 -> Mux1/2  "Pitch Rate"
  Gain5/1 -> Mux1/3  "Yaw Rate"
  Mux1/1 -> Reshape1/1
  Matrix Multiply/1 -> Scope 2/1, Bus Creator/1  "eulerAngles"
  Matrix Multiply1/1 -> Scope 1/1, Bus Creator/2  "gyroRates"
  Reshape/1 -> Matrix Multiply/2
  [DcM] -> Matrix Multiply/1
  Reshape1/1 -> Matrix Multiply1/2
  [DcM] -> Matrix Multiply1/1
  Demux/3 -> Display2/1
  Demux/2 -> Display3/1
  Demux/1 -> Display4/1

== system towTest_dualWinch/Serial CMD/deg-to-us ==
  In1 : Inport
  Constant1 : Constant  Value=1500
  Gain : Gain  Gain=10
  Sum : Sum  Inputs=|++
  Out1 : Outport
  wires:
  Gain/1 -> Sum/1
  Constant1/1 -> Sum/2
  In1/1 -> Gain/1
  Sum/1 -> Out1/1

== system towTest_dualWinch/Serial CMD/deg-to-us1 ==
  pitchCMD : Inport
  Constant1 : Constant  Value=1500
  Gain : Gain  Gain=10
  Sum : Sum  Inputs=|++
  Out1 : Outport
  wires:
  Sum/1 -> Out1/1
  pitchCMD/1 -> Gain/1
  Constant1/1 -> Sum/2
  Gain/1 -> Sum/1

== system towTest_dualWinch/Serial CMD/deg-to-us2 ==
  In1 : Inport
  Constant1 : Constant  Value=1500
  Gain : Gain  Gain=10
  Sum : Sum  Inputs=|++
  Out1 : Outport
  wires:
  Gain/1 -> Sum/1
  Constant1/1 -> Sum/2
  In1/1 -> Gain/1
  Sum/1 -> Out1/1

== system towTest_dualWinch/Serial CMD/to2uint1 ==
  " " : Inport
  Bit Packing 1 : xpcutilitieslib/Bit Packing   MaskBitPatterns={[0:7]}  MaskPackDataType=uint8  MaskPackDataSize=[1]
      settings: SourceProductBaseCode=XP
  Bit Packing 2 : xpcutilitieslib/Bit Packing   MaskBitPatterns={[0:7]}  MaskPackDataType=uint8  MaskPackDataSize=[1]
      settings: SourceProductBaseCode=XP
  Bit Shift2 : hdlsllib/Logic and Bit Operations/Bit Shift  mode=Shift Right Arithmetic  N=8
  Cast4 : DataTypeConversion  OutDataTypeStr=uint16
  Out1 : Outport
  Out2 : Outport  Port=2
  wires:
  Bit Packing 1/1 -> Out1/1
  " "/1 -> Cast4/1
  Cast4/1 -> Bit Packing 1/1, Bit Shift2/1
  Bit Packing 2/1 -> Out2/1
  Bit Shift2/1 -> Bit Packing 2/1

== system towTest_dualWinch/Serial CMD/to2uint2 ==
  " " : Inport
  Bit Packing 1 : xpcutilitieslib/Bit Packing   MaskBitPatterns={[0:7]}  MaskPackDataType=uint8  MaskPackDataSize=[1]
      settings: SourceProductBaseCode=XP
  Bit Packing 2 : xpcutilitieslib/Bit Packing   MaskBitPatterns={[0:7]}  MaskPackDataType=uint8  MaskPackDataSize=[1]
      settings: SourceProductBaseCode=XP
  Bit Shift2 : hdlsllib/Logic and Bit Operations/Bit Shift  mode=Shift Right Arithmetic  N=8
  Cast4 : DataTypeConversion  OutDataTypeStr=uint16
  Out1 : Outport
  Out2 : Outport  Port=2
  wires:
  Bit Shift2/1 -> Bit Packing 2/1
  Bit Packing 2/1 -> Out2/1
  Cast4/1 -> Bit Shift2/1, Bit Packing 1/1
  " "/1 -> Cast4/1
  Bit Packing 1/1 -> Out1/1

== system towTest_dualWinch/Serial CMD/to2uint8 ==
  " " : Inport
  Bit Packing 1 : xpcutilitieslib/Bit Packing   MaskBitPatterns={[0:7]}  MaskPackDataType=uint8  MaskPackDataSize=[1]
      settings: SourceProductBaseCode=XP
  Bit Packing 2 : xpcutilitieslib/Bit Packing   MaskBitPatterns={[0:7]}  MaskPackDataType=uint8  MaskPackDataSize=[1]
      settings: SourceProductBaseCode=XP
  Bit Shift2 : hdlsllib/Logic and Bit Operations/Bit Shift  mode=Shift Right Arithmetic  N=8
  Cast4 : DataTypeConversion  OutDataTypeStr=uint16
  Out1 : Outport
  Out2 : Outport  Port=2
  wires:
  Bit Shift2/1 -> Bit Packing 2/1
  Cast4/1 -> Bit Shift2/1, Bit Packing 1/1
  " "/1 -> Cast4/1
  Bit Packing 1/1 -> Out1/1
  Bit Packing 2/1 -> Out2/1

== system towTest_dualWinch/Serial Unpacking/Subsystem ==
  In1 : Inport
  In2 : Inport  Port=2
  "Bit Packing " : xpcutilitieslib/Bit Packing   MaskBitPatterns={[0:15]}  MaskPackDataType=uint16  MaskPackDataSize=[1]
      settings: SourceProductBaseCode=XP
  Bit Packing 3 : xpcutilitieslib/Bit Packing   MaskBitPatterns={[0:7]}  MaskPackDataType=uint32  MaskPackDataSize=[1]
      settings: SourceProductBaseCode=XP
  Bit Packing 4 : xpcutilitieslib/Bit Packing   MaskBitPatterns={[0:7]}  MaskPackDataType=uint32  MaskPackDataSize=[1]
      settings: SourceProductBaseCode=XP
  Bit Shift3 : hdlsllib/Logic and Bit Operations/Bit Shift  mode=Shift Left Logical  N=8
  Bitwise Operator : simulink/Logic and Bit Operations/Bitwise Operator  logicop=OR  UseBitMask=off  NumInputPorts=2  BitMask=bin2dec('00000000')  BitMaskRealWorld=Stored Integer
  Cast To Double1 : DataTypeConversion  OutDataTypeStr=double
  Double : Outport
  wires:
  In1/1 -> Bit Packing 3/1
  Cast To Double1/1 -> Double/1
  Bit Packing 3/1 -> Bit Shift3/1
  Bit Packing 4/1 -> Bitwise Operator/2
  In2/1 -> Bit Packing 4/1
  Bitwise Operator/1 -> "Bit Packing "/1
  "Bit Packing "/1 -> Cast To Double1/1
  Bit Shift3/1 -> Bitwise Operator/1

== system towTest_dualWinch/Serial Unpacking/Subsystem1 ==
  In1 : Inport
  In2 : Inport  Port=2
  "Bit Packing " : xpcutilitieslib/Bit Packing   MaskBitPatterns={[0:15]}  MaskPackDataType=uint16  MaskPackDataSize=[1]
      settings: SourceProductBaseCode=XP
  Bit Packing 3 : xpcutilitieslib/Bit Packing   MaskBitPatterns={[0:7]}  MaskPackDataType=uint32  MaskPackDataSize=[1]
      settings: SourceProductBaseCode=XP
  Bit Packing 4 : xpcutilitieslib/Bit Packing   MaskBitPatterns={[0:7]}  MaskPackDataType=uint32  MaskPackDataSize=[1]
      settings: SourceProductBaseCode=XP
  Bit Shift3 : hdlsllib/Logic and Bit Operations/Bit Shift  mode=Shift Left Logical  N=8
  Bitwise Operator : simulink/Logic and Bit Operations/Bitwise Operator  logicop=OR  UseBitMask=off  NumInputPorts=2  BitMask=bin2dec('00000000')  BitMaskRealWorld=Stored Integer
  Cast To Double1 : DataTypeConversion  OutDataTypeStr=double
  Double : Outport
  wires:
  In1/1 -> Bit Packing 3/1
  Cast To Double1/1 -> Double/1
  Bit Packing 3/1 -> Bit Shift3/1
  Bit Packing 4/1 -> Bitwise Operator/2
  In2/1 -> Bit Packing 4/1
  Bitwise Operator/1 -> "Bit Packing "/1
  "Bit Packing "/1 -> Cast To Double1/1
  Bit Shift3/1 -> Bitwise Operator/1

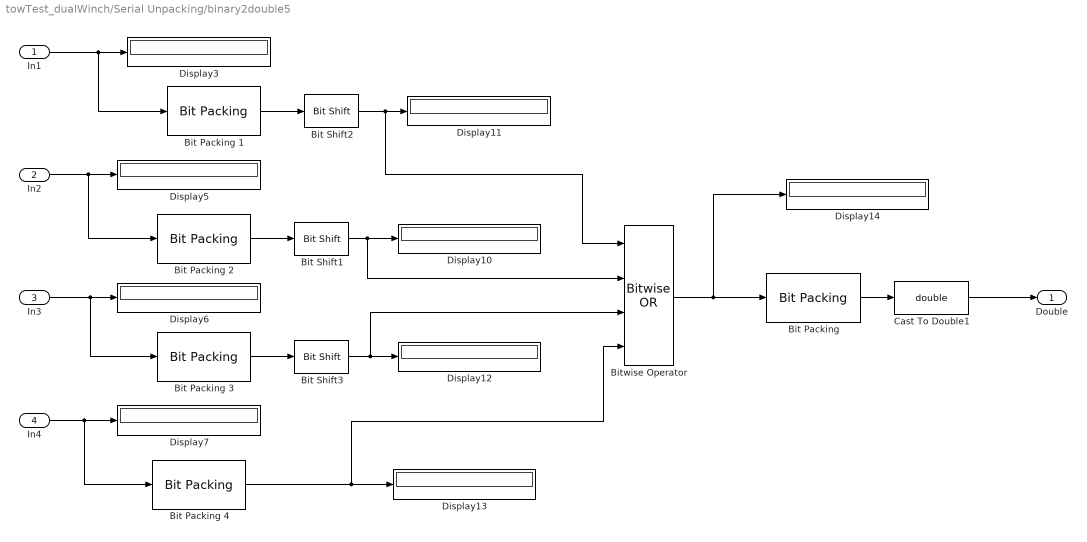
== system towTest_dualWinch/Serial Unpacking/binary2double5 ==
  In1 : Inport
  In2 : Inport  Port=2
  In3 : Inport  Port=3
  In4 : Inport  Port=4
  Bit Packing {,1..4} (5 alike) : xpcutilitieslib/Bit Packing 
      settings: SourceProductBaseCode=XP
  Bit Shift1 : hdlsllib/Logic and Bit Operations/Bit Shift  mode=Shift Left Logical  N=16
  Bit Shift2 : hdlsllib/Logic and Bit Operations/Bit Shift  mode=Shift Left Logical  N=24
  Bit Shift3 : hdlsllib/Logic and Bit Operations/Bit Shift  mode=Shift Left Logical  N=8
  Bitwise Operator : simulink/Logic and Bit Operations/Bitwise Operator  logicop=OR  UseBitMask=off  NumInputPorts=4  BitMask=bin2dec('00000000')  BitMaskRealWorld=Stored Integer
  Cast To Double1 : DataTypeConversion  OutDataTypeStr=double
  Display{3,5..7,10..14} (9 alike) : Display
      settings: Format=hex (Stored Integer)
  Double : Outport
  wires:
  Bit Shift1/1 -> Bitwise Operator/2, Display10/1
  Bitwise Operator/1 -> Display14/1, "Bit Packing "/1
  Bit Packing 1/1 -> Bit Shift2/1
  Bit Packing 4/1 -> Bitwise Operator/4, Display13/1
  In1/1 -> Bit Packing 1/1, Display3/1
  In3/1 -> Bit Packing 3/1, Display6/1
  Bit Shift2/1 -> Bitwise Operator/1, Display11/1
  Bit Packing 2/1 -> Bit Shift1/1
  "Bit Packing "/1 -> Cast To Double1/1
  Bit Shift3/1 -> Bitwise Operator/3, Display12/1
  Bit Packing 3/1 -> Bit Shift3/1
  In2/1 -> Bit Packing 2/1, Display5/1
  In4/1 -> Bit Packing 4/1, Display7/1
  Cast To Double1/1 -> Double/1

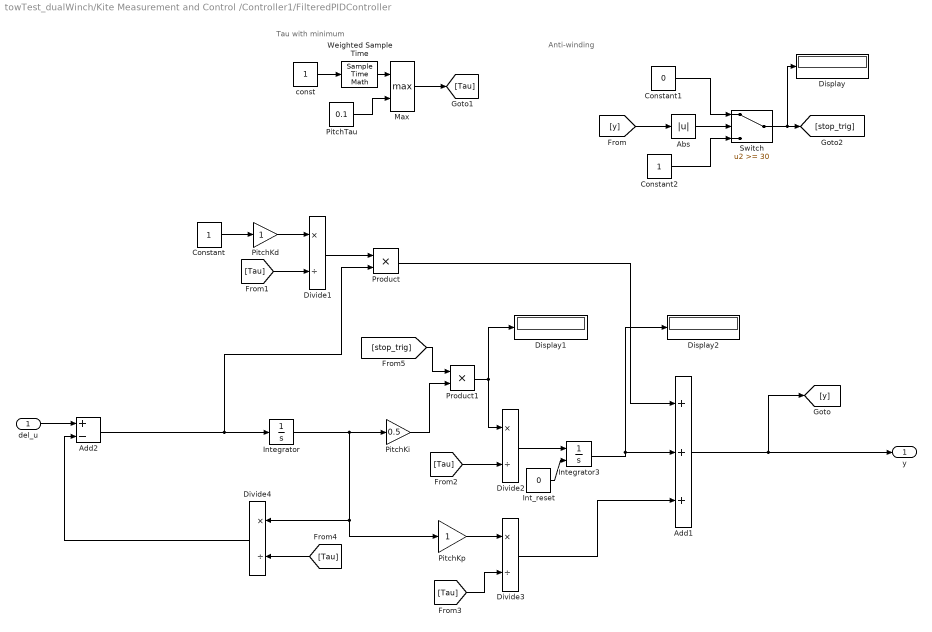
== system towTest_dualWinch/Kite Measurement and Control /Controller1/FilteredPIDController ==
  note: Anti-winding
  note: Tau with minimum
  del_u : Inport
  Abs : Abs
  Add1 : Sum  Inputs=+++
  Add2 : Sum  Inputs=+-
  Constant : Constant
  Constant1 : Constant  Value=0
  Constant2 : Constant
  Display : Display
  Display1 : Display
  Display2 : Display
  Divide{1..4} (4 alike) : Product  Inputs=*/
  Int_reset : Constant  Value=0
  Integrator : Integrator
  Integrator3 : Integrator  ExternalReset=either
  Max : MinMax  Function=max  Inputs=2
  PitchKd : Gain
  PitchKi : Gain  Gain=0.5
  PitchKp : Gain
  PitchTau : Constant  Value=0.1
  Product : Product
  Product1 : Product
  Switch : Switch  Threshold=30
  Weighted Sample Time : SampleTimeMath  TsampMathOp=Ts Only
  const : Constant
  y : Outport
  wires:
  PitchTau/1 -> Max/2
  Add1/1 -> [y], y/1
  const/1 -> Weighted Sample Time/1
  Weighted Sample Time/1 -> Max/1
  Max/1 -> [Tau]
  PitchKd/1 -> Divide1/1
  Constant/1 -> PitchKd/1
  [Tau] -> Divide1/2
  Divide1/1 -> Product/1
  Integrator/1 -> PitchKp/1, Divide4/1, PitchKi/1
  [Tau] -> Divide2/2
  Divide2/1 -> Integrator3/1
  Integrator3/1 -> Display2/1, Add1/2
  Product/1 -> Add1/1
  PitchKp/1 -> Divide3/1
  Divide3/1 -> Add1/3
  [Tau] -> Divide3/2
  [Tau] -> Divide4/2
  del_u/1 -> Add2/1
  Divide4/1 -> Add2/2
  Add2/1 -> Product/2, Integrator/1
  [y] -> Abs/1
  Abs/1 -> Switch/2
  Constant1/1 -> Switch/1
  Constant2/1 -> Switch/3
  Switch/1 -> Display/1, [stop_trig]
  PitchKi/1 -> Product1/2
  [stop_trig] -> Product1/1
  Product1/1 -> Divide2/1, Display1/1
  Int_reset/1 -> Integrator3/2

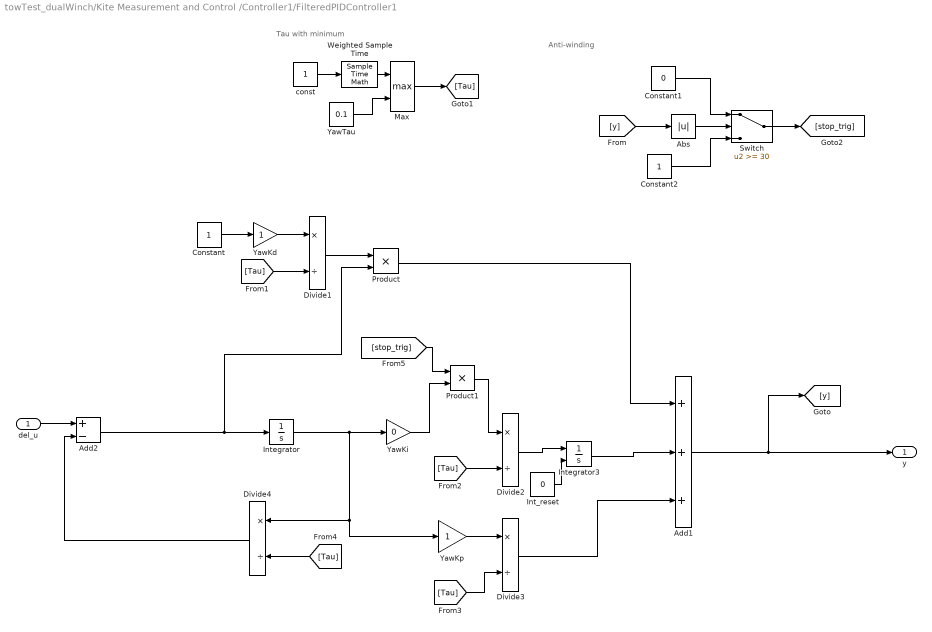
== system towTest_dualWinch/Kite Measurement and Control /Controller1/FilteredPIDController1 ==
  note: Anti-winding
  note: Tau with minimum
  del_u : Inport
  Abs : Abs
  Add1 : Sum  Inputs=+++
  Add2 : Sum  Inputs=+-
  Constant : Constant
  Constant1 : Constant  Value=0
  Constant2 : Constant
  Divide{1..4} (4 alike) : Product  Inputs=*/
  Int_reset : Constant  Value=0
  Integrator : Integrator
  Integrator3 : Integrator  ExternalReset=either
  Max : MinMax  Function=max  Inputs=2
  Product : Product
  Product1 : Product
  Switch : Switch  Threshold=30
  Weighted Sample Time : SampleTimeMath  TsampMathOp=Ts Only
  YawKd : Gain
  YawKi : Gain  Gain=0
  YawKp : Gain
  YawTau : Constant  Value=0.1
  const : Constant
  y : Outport
  wires:
  YawTau/1 -> Max/2
  Add1/1 -> [y], y/1
  const/1 -> Weighted Sample Time/1
  Weighted Sample Time/1 -> Max/1
  Max/1 -> [Tau]
  YawKd/1 -> Divide1/1
  Constant/1 -> YawKd/1
  [Tau] -> Divide1/2
  Divide1/1 -> Product/1
  Integrator/1 -> YawKp/1, Divide4/1, YawKi/1
  [Tau] -> Divide2/2
  Divide2/1 -> Integrator3/1
  Integrator3/1 -> Add1/2
  Product/1 -> Add1/1
  YawKp/1 -> Divide3/1
  Divide3/1 -> Add1/3
  [Tau] -> Divide3/2
  [Tau] -> Divide4/2
  del_u/1 -> Add2/1
  Divide4/1 -> Add2/2
  Add2/1 -> Product/2, Integrator/1
  [y] -> Abs/1
  Abs/1 -> Switch/2
  Constant1/1 -> Switch/1
  Constant2/1 -> Switch/3
  Switch/1 -> [stop_trig]
  YawKi/1 -> Product1/2
  [stop_trig] -> Product1/1
  Product1/1 -> Divide2/1
  Int_reset/1 -> Integrator3/2

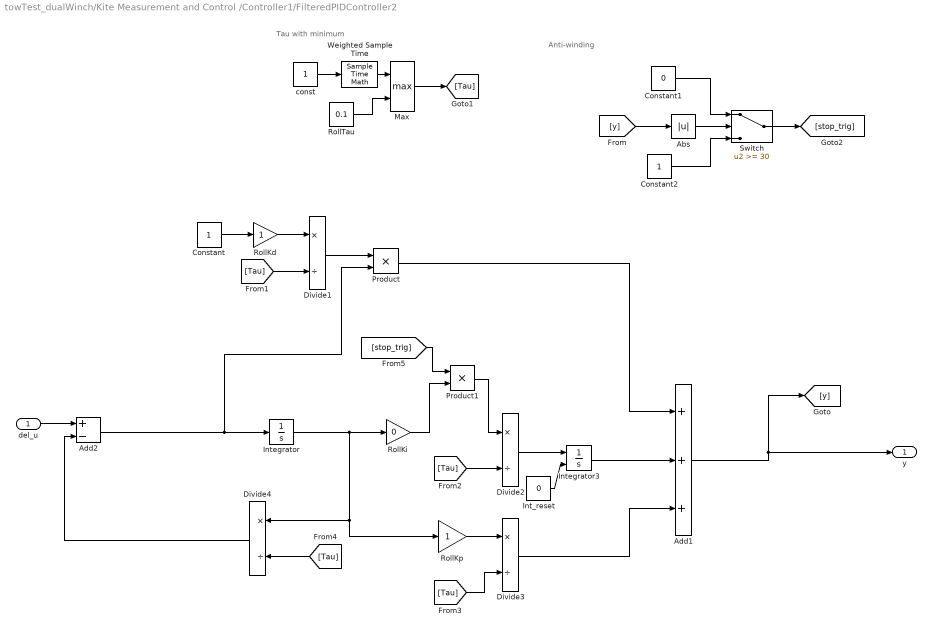
== system towTest_dualWinch/Kite Measurement and Control /Controller1/FilteredPIDController2 ==
  note: Tau with minimum
  note: Anti-winding
  del_u : Inport
  Abs : Abs
  Add1 : Sum  Inputs=+++
  Add2 : Sum  Inputs=+-
  Constant : Constant
  Constant1 : Constant  Value=0
  Constant2 : Constant
  Divide{1..4} (4 alike) : Product  Inputs=*/
  Int_reset : Constant  Value=0
  Integrator : Integrator
  Integrator3 : Integrator  ExternalReset=either
  Max : MinMax  Function=max  Inputs=2
  Product : Product
  Product1 : Product
  RollKd : Gain
  RollKi : Gain  Gain=0
  RollKp : Gain
  RollTau : Constant  Value=0.1
  Switch : Switch  Threshold=30
  Weighted Sample Time : SampleTimeMath  TsampMathOp=Ts Only
  const : Constant
  y : Outport
  wires:
  Product1/1 -> Divide2/1
  [stop_trig] -> Product1/1
  RollKi/1 -> Product1/2
  Switch/1 -> [stop_trig]
  Constant2/1 -> Switch/3
  Constant1/1 -> Switch/1
  Abs/1 -> Switch/2
  [y] -> Abs/1
  Add2/1 -> Integrator/1, Product/2
  Divide4/1 -> Add2/2
  del_u/1 -> Add2/1
  [Tau] -> Divide4/2
  [Tau] -> Divide3/2
  Divide3/1 -> Add1/3
  RollKp/1 -> Divide3/1
  Product/1 -> Add1/1
  Integrator3/1 -> Add1/2
  Divide2/1 -> Integrator3/1
  [Tau] -> Divide2/2
  Integrator/1 -> RollKi/1, Divide4/1, RollKp/1
  Divide1/1 -> Product/1
  [Tau] -> Divide1/2
  Constant/1 -> RollKd/1
  RollKd/1 -> Divide1/1
  Max/1 -> [Tau]
  Weighted Sample Time/1 -> Max/1
  const/1 -> Weighted Sample Time/1
  Add1/1 -> y/1, [y]
  RollTau/1 -> Max/2
  Int_reset/1 -> Integrator3/2

== system towTest_dualWinch/Kite Measurement and Control /Controller1/FilteredPIDController_Pitchold ==
  del_u : Inport
  Add : Sum  Inputs=+-
  Add1 : Sum  Inputs=+++
  Divide : Product  Inputs=*/
  Integrator : Integrator
  Integrator1 : Integrator
  Integrator2 : Integrator
  Max : MinMax  Function=max  Inputs=2
  PitchKd : Gain
  PitchKi : Gain  Gain=0
  PitchKp : Gain
  PitchTau : Constant  Value=0.1
  Weighted Sample Time : SampleTimeMath  TsampMathOp=Ts Only
  const : Constant
  y : Outport
  wires:
  PitchTau/1 -> Max/2
  Divide/1 -> y/1, [y]
  Add/1 -> Integrator/1
  const/1 -> Weighted Sample Time/1
  Integrator/1 -> Add1/1
  Integrator1/1 -> Integrator2/1
  [y] -> Add/2
  Max/1 -> Divide/2
  PitchKd/1 -> Add1/3
  Add1/1 -> Divide/1
  PitchKi/1 -> Integrator1/1
  PitchKp/1 -> Add/1
  Weighted Sample Time/1 -> Max/1
  Integrator2/1 -> Add1/2
  del_u/1 -> PitchKd/1, PitchKi/1, PitchKp/1

== system towTest_dualWinch/Kite Measurement and Control /Controller1/FilteredPIDController_oldRoll ==
  del_u : Inport
  Add : Sum  Inputs=+-
  Add1 : Sum  Inputs=+++
  Divide : Product  Inputs=*/
  Integrator : Integrator
  Integrator1 : Integrator
  Integrator2 : Integrator
  Max : MinMax  Function=max  Inputs=2
  RollKd : Gain
  RollKi : Gain  Gain=0
  RollKp : Gain
  RollTau : Constant  Value=0.1
  Weighted Sample Time : SampleTimeMath  TsampMathOp=Ts Only
  const : Constant
  y : Outport
  wires:
  RollTau/1 -> Max/2
  Divide/1 -> y/1, [y]
  Add/1 -> Integrator/1
  const/1 -> Weighted Sample Time/1
  Integrator/1 -> Add1/1
  Integrator1/1 -> Integrator2/1
  [y] -> Add/2
  Max/1 -> Divide/2
  RollKd/1 -> Add1/3
  Add1/1 -> Divide/1
  RollKi/1 -> Integrator1/1
  RollKp/1 -> Add/1
  Weighted Sample Time/1 -> Max/1
  Integrator2/1 -> Add1/2
  del_u/1 -> RollKd/1, RollKi/1, RollKp/1

== system towTest_dualWinch/Kite Measurement and Control /Controller1/FilteredPIDController_oldYaw ==
  del_u : Inport
  Add : Sum  Inputs=+-
  Add1 : Sum  Inputs=+++
  Divide : Product  Inputs=*/
  Integrator : Integrator
  Integrator1 : Integrator
  Integrator2 : Integrator
  Max : MinMax  Function=max  Inputs=2
  Weighted Sample Time : SampleTimeMath  TsampMathOp=Ts Only
  YawKd : Gain  Gain=0.2
  YawKi : Gain  Gain=0.3
  YawKp : Gain  Gain=0.1
  YawTau : Constant  Value=0.4
  const : Constant
  y : Outport
  wires:
  YawTau/1 -> Max/2
  Divide/1 -> y/1, [y]
  Add/1 -> Integrator/1
  const/1 -> Weighted Sample Time/1
  Integrator/1 -> Add1/1
  Integrator1/1 -> Integrator2/1
  [y] -> Add/2
  Max/1 -> Divide/2
  YawKd/1 -> Add1/3
  Add1/1 -> Divide/1
  YawKi/1 -> Integrator1/1
  YawKp/1 -> Add/1
  Weighted Sample Time/1 -> Max/1
  Integrator2/1 -> Add1/2
  del_u/1 -> YawKd/1, YawKi/1, YawKp/1
